simulink library "EngineSystemSubmodel"  (Simulink 8.1)
settings: Solver=ode45  StartTime=0.0  StopTime=10.0  FixedStep=1e-4  RelTol=1e-3
values from neighbouring files (symbols this model uses):
  B = [B1;B2]    [GensetRespOptimiztion.m]    (also in GensetRespOptimiztionTorstein.m; Init8RTFLEX68D.m = 0.68; init_MVM.m = 0.127)
  beta = 0.75    [Init8RTFLEX68D.m]
  cAStartRef = 104.8    [Init8RTFLEX68D.m]
  coeffMechEff = [0.135;0.155]    [Init8RTFLEX68D.m]
  comp_eff_map = [0 0 0 0 0 0 0 0 0 0 0 0 ... (250000 elements, 500x500)]    [comp_map.mat]    (also in comp_mapABB A175-35L.mat)
  comp_flow_map = [0 0 0 0 0 0 0 0 0 0 0 0 ... (250000 elements, 500x500)]    [comp_map.mat]    (also in comp_mapABB A175-35L.mat)
  D_turb_wheel = TC.TC_map.turb.D_wheel    [init_MVM.m]
  dCALiftDown = cAVVDownRef(end) - cAVVDownRef(1)    [Init8RTFLEX68D.m]
  dCALiftTopRef = 63.5    [Init8RTFLEX68D.m]
  dCALiftUp = cAVVUpRef(end) - cAVVUpRef(1)    [Init8RTFLEX68D.m]
  Dp = 0.383    [Init8RTFLEX68D.m]
  Ds = 0.079    [Init8RTFLEX68D.m]
  Dv = 0.425    [Init8RTFLEX68D.m]
  eff_coeff = [-1.0889528323728;0.91854258409396;-0.10659748546926;                     0.21229452390244;-0.053186221596493;-0.005451194709834]    [Init8RTFLEX68D.m]
  eta_turb_max = TC.TC_map.turb.eff_max    [init_MVM.m]
  flow_coeff_turb = [-1.585326540339;-4.823836967181;1.5853156139822]    [Init8RTFLEX68D.m]    (also in init_MVM.m = TC.TC_map.turb.flow_fit_coeff)
  fs = 0.0683    [Init8RTFLEX68D.m]    (also in NOxProcessGUI.m = varargin{2}; initHybrid.m; initMV.m; init_MVM.m = 0.0682925799315)
  genset = generators(1)    [runTempCyl4S.m]
  J_tc = TC.SAE_map_comp.inertia    [init_MVM.m]
  jShaft = 0    [EngineSystemParameters.m]    (also in Init8RTFLEX68D.m = 323000)
  jTC = 2    [Init8RTFLEX68D.m]
  Kb = 1*ones(engines,1)    [initHybrid.m]    (also in initMV.m; init_MVM.m = 1; init_ele.m = 1)
  Kd = 20*ones(engines,1)    [initHybrid.m]    (also in initMV.m; init_MVM.m = 10; init_ele.m = 20)
  Ki = 20*ones(engines,1)    [initHybrid.m]    (also in initMV.m; init_MVM.m = 10; init_ele.m = 20)
  Kp = 20*ones(engines,1)    [initHybrid.m]    (also in initMV.m; init_MVM.m = 10; init_ele.m = 20)
  lambdaCrank = 0.5056    [Init8RTFLEX68D.m]
  liftMax = 0.17    [Init8RTFLEX68D.m]
  Load_amp = x(4) + xRef(i)    [GetErrGensetResp.m]    (also in runsimulation.m = 0.55; runsimulationRecovery.m = InitialLoad(jj) + LoadStep(ii))
  Load_bias = x(4)    [GetErrGensetResp.m]    (also in runsimulation.m = 0.15; runsimulationRecovery.m = InitialLoad(jj))
  Load_index = 1    [GetErrGensetResp.m]    (also in runsimulation.m; runsimulationRecovery.m)
  mqfCycMax = 9.5547e-2    (= 0.095547)    [Init8RTFLEX68D.m]
  N = x*noMol    [NOxProcessGUI.m]    (also in initHybrid.m = .1*ones(engines,1); initMV.m = .1*ones(engines,1); init_ele.m = 0.1)
  n288_rep = [0 222.054 444.108 666.162 888.216 1110.27 1332.324 1554.378 1776.432 1998.486 2220.54 2442.594 ... (500 elements, 1x500)]    [comp_map.mat]
  nPort = 28    [Init8RTFLEX68D.m]
  npr = length(pr_rep)    [Init8RTFLEX68D.m]    (also in initHybrid.m; initMV.m; init_MVM.m)
  nsp = length(n288_rep)    [Init8RTFLEX68D.m]    (also in initHybrid.m; initMV.m; init_MVM.m)
  nStroke = 2    [Init8RTFLEX68D.m]
  omegat0 = RPM_TC_initial/30*pi    [init_MVM.m]
  pr_rep = [1.01 1.0150249672 1.0200499344 1.0250749016 1.0300998688 1.035124836 1.0401498032 1.0451747704 1.0501997376 1.0552247048 1.060249672 1.0652746392 ... (500 elements, 1x500)]    [comp_map.mat]
  r = 0.035    [Init8RTFLEX68D.m]
  Start_time = 50    [GetErrGensetResp.m]    (also in runsimulation.m; runsimulationRecovery.m)
  stroke = 2.72    [Init8RTFLEX68D.m]
  T_load = 1    [GetErrGensetResp.m]    (also in runsimulation.m; runsimulationRecovery.m)
  T_ref_turb = TC.TC_map.turb.T_ref    [init_MVM.m]
  u0 = 0.2    [init_MVM.m]
  Uc_opt = TC.TC_map.turb.Uc_opt    [init_MVM.m]
  w = 0.021    [Init8RTFLEX68D.m]
  wasteGateMax = 10    [Init8RTFLEX68D.m]
  wasteGateMin = 0    [Init8RTFLEX68D.m]
  wiebePara = [0.07;0.57;3.05;11;24;56.3;1.5;1;0.7]    [Init8RTFLEX68D.m]
  X = 0.07    [Init8RTFLEX68D.m]
  Y = 0.16    [Init8RTFLEX68D.m]
undefined symbols (not defined in the file or in its folder): aCrank, cAVVDownRef, cAVVUpRef, liftDownRef, liftUpRef, omega0, Td, Ti, u_max
undefined symbols (not defined in the file): BWdmExhBypass, cAlpha, cCylHT, E0A, ECyl0, hn, KbWG, KpWG, lowerCloseSPWG, m0A, mb0A, mbCyl0, mCp, mCyl0, nCyl, phi0, phi0A, phi0rad, RPM0, RPMMax, RPMT0, TiWG, upperOpenWG, V0A, vCyl0, wasteGateRatio
libraries: EngineSystemSubmodel x49, simulink x1
(part 3 of 3)

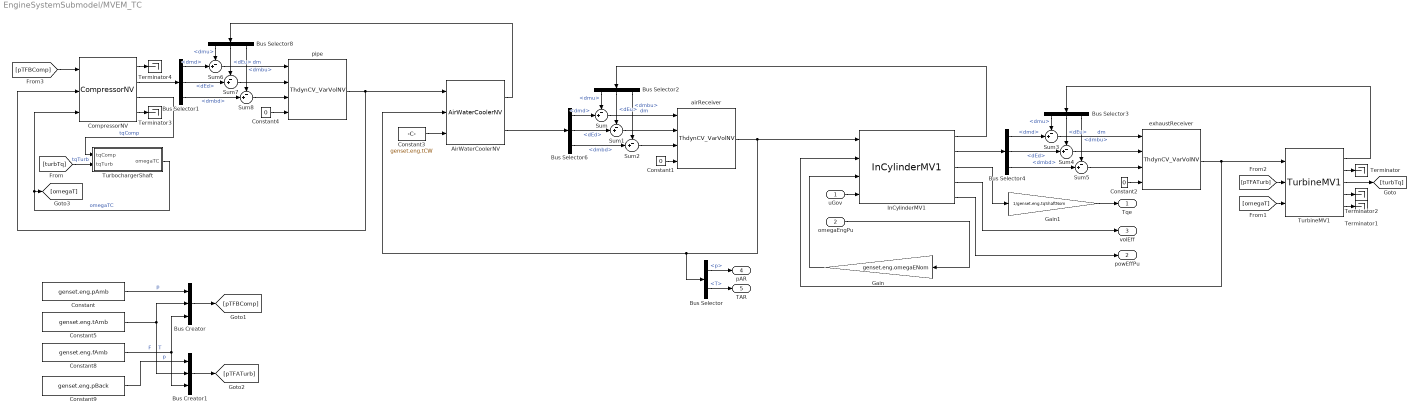
== system EngineSystemSubmodel/MVEM_TC ==
  uGov : Inport
  omegaEngPu : Inport  Port=2
  AirWaterCoolerNV : EngineSystemSubmodel/AirWaterCoolerNV  fs=genset.eng.fs  Cd=genset.eng.cdCool  A_air_path=genset.eng.aAirPath  dm_cw=genset.eng.dmCW  coeff_T_cw_K=genset.eng.coeffKTCW  Cp_cw=genset.eng.cpCW  D_cw_pipe=genset.eng.dPipeCW
  Bus Creator : BusCreator  Inputs=3
  Bus Creator1 : BusCreator  Inputs=3
  Bus Selector : BusSelector  OutputSignals=p,T
  Bus Selector1 : BusSelector  OutputSignals=dmd,dEd,dmbd
  Bus Selector2 : BusSelector  OutputSignals=dmu,dEu,dmbu
  Bus Selector3 : BusSelector  OutputSignals=dmu,dEu,dmbu
  Bus Selector4 : BusSelector  OutputSignals=dmd,dEd,dmbd
  Bus Selector6 : BusSelector  OutputSignals=dmd,dEd,dmbd
  Bus Selector8 : BusSelector  OutputSignals=dmu,dEu,dmbu
  CompressorNV : EngineSystemSubmodel/CompressorNV  fs=genset.eng.fs  comp_flow_map=genset.eng.compFlowMap  comp_eff_map=genset.eng.compEffMap  pr_rep=genset.eng.prRep  n288_rep=genset.eng.n288Rep  npr=genset.eng.npr  nsp=genset.eng.nsp
  Constant : Constant  Value=genset.eng.pAmb
  Constant1 : Constant  Value=0
  Constant2 : Constant  Value=0
  Constant3 : Constant  Value=genset.eng.tCW
  Constant4 : Constant  Value=0
  Constant5 : Constant  Value=genset.eng.tAmb
  Constant8 : Constant  Value=genset.eng.fAmb
  Constant9 : Constant  Value=genset.eng.pBack
  Gain : Gain  Gain=genset.eng.omegaENom
  Gain1 : Gain  Gain=1/genset.eng.tqShaftNom
  InCylinderMV1 : EngineSystemSubmodel/InCylinderMV1  fs=genset.eng.fs  Vd=genset.eng.vD  LHV=genset.eng.LHV  Pe_nom=genset.eng.powNom  SFC=genset.eng.SFC  vol_eff_coeff1=genset.eng.volEff1  vol_eff_coeff2=genset.eng.volEff2  T_pe=genset.eng.tPe  nstroke=genset.eng.nStroke  m_f_cyc_max=genset.eng.mFCycMax  C1=genset.eng.C1  p_a_inf=genset.eng.pAInf  Pe0=genset.eng.powL0*genset.eng.powNom
  Sum{,1..8} (9 alike) : Sum  Inputs=-+|
  Terminator{,1..4} (5 alike) : Terminator
  TurbineMV1 : EngineSystemSubmodel/TurbineMV1  fs=genset.eng.fs  flow_coeff_turb=genset.eng.flowCoeffTurb  D_turb_wheel=genset.eng.dTurbWheel  Uc_opt=genset.eng.ucOpt  eta_turb_max=genset.eng.effTurbMax  T_ref_turb=genset.eng.T_ref_turb
  TurbochargerShaft : Subsystem
  airReceiver : EngineSystemSubmodel/ThdynCV_VarVolNV  fs=genset.eng.fs  m0=genset.eng.m0AR  E0=genset.eng.E0AR  mb0=genset.eng.mb0AR  V0=genset.eng.vAR
  exhaustReceiver : EngineSystemSubmodel/ThdynCV_VarVolNV  fs=genset.eng.fs  m0=genset.eng.m0ER  E0=genset.eng.E0ER  mb0=genset.eng.mb0ER  V0=genset.eng.vER
  pipe : EngineSystemSubmodel/ThdynCV_VarVolNV  fs=genset.eng.fs  m0=genset.eng.m0PipeAComp  E0=genset.eng.e0PipeAComp  mb0=genset.eng.mb0PipeAComp  V0=genset.eng.vPipeAComp
  Tqe : Outport
  powEffPu : Outport  Port=2
  volEff : Outport  Port=3
  pAR : Outport  Port=4
  TAR : Outport  Port=5
  wires:
  TurbineMV1/2 -> Terminator/1
  TurbineMV1/4 -> Terminator2/1
  TurbineMV1/5 -> Terminator1/1
  Constant5/1 -> Bus Creator1/2, Bus Creator/2  "T"
  Constant8/1 -> Bus Creator1/3, Bus Creator/3  "F"
  Constant/1 -> Bus Creator/1  "p"
  Bus Creator1/1 -> [pTFATurb]
  Constant9/1 -> Bus Creator1/1  "p"
  Bus Selector3/2 -> Sum4/1  "<dEu>"
  [pTFBComp] -> CompressorNV/1
  [pTFATurb] -> TurbineMV1/2
  TurbineMV1/3 -> [turbTq]
  Bus Selector3/3 -> Sum5/1  "<dmbu>"
  InCylinderMV1/1 -> Bus Selector2/1
  Bus Selector2/1 -> Sum/1  "<dmu>"
  Sum/1 -> airReceiver/1  "dm"
  Bus Selector2/2 -> Sum1/1  "<dEu>"
  Bus Selector2/3 -> Sum2/1  "<dmbu>"
  exhaustReceiver/1 -> TurbineMV1/1, InCylinderMV1/2
  omegaEngPu/1 -> Gain/1
  airReceiver/1 -> InCylinderMV1/1, Bus Selector/1, AirWaterCoolerNV/2
  Constant4/1 -> pipe/4
  Bus Selector1/2 -> Sum7/2  "<dEd>"
  Bus Selector1/3 -> Sum8/2  "<dmbd>"
  Bus Selector1/1 -> Sum6/2  "<dmd>"
  Bus Creator/1 -> [pTFBComp]
  Bus Selector3/1 -> Sum3/1  "<dmu>"
  [omegaT] -> TurbineMV1/3
  TurbineMV1/1 -> Bus Selector3/1
  InCylinderMV1/5 -> powEffPu/1
  Sum6/1 -> pipe/1  "dm"
  AirWaterCoolerNV/2 -> Bus Selector6/1
  Bus Selector8/2 -> Sum7/1  "<dEu>"
  Sum7/1 -> pipe/2
  Bus Selector8/1 -> Sum6/1  "<dmu>"
  Gain/1 -> InCylinderMV1/3
  Sum8/1 -> pipe/3
  pipe/1 -> CompressorNV/2, AirWaterCoolerNV/1
  Bus Selector8/3 -> Sum8/1  "<dmbu>"
  AirWaterCoolerNV/1 -> Bus Selector8/1
  Bus Selector6/1 -> Sum/2  "<dmd>"
  Bus Selector6/2 -> Sum1/2  "<dEd>"
  Sum3/1 -> exhaustReceiver/1  "dm"
  Constant2/1 -> exhaustReceiver/4
  Sum5/1 -> exhaustReceiver/3
  Sum1/1 -> airReceiver/2
  Sum2/1 -> airReceiver/3
  Bus Selector4/2 -> Sum4/2  "<dEd>"
  Sum4/1 -> exhaustReceiver/2
  InCylinderMV1/2 -> Bus Selector4/1
  Bus Selector6/3 -> Sum2/2  "<dmbd>"
  Bus Selector4/3 -> Sum5/2  "<dmbd>"
  Constant1/1 -> airReceiver/4
  Bus Selector4/1 -> Sum3/2  "<dmd>"
  CompressorNV/2 -> Bus Selector1/1
  Constant3/1 -> AirWaterCoolerNV/3
  InCylinderMV1/4 -> volEff/1
  uGov/1 -> InCylinderMV1/4
  Gain1/1 -> Tqe/1
  Bus Selector/1 -> pAR/1  "<p>"
  Bus Selector/2 -> TAR/1  "<T>"
  CompressorNV/4 -> Terminator3/1
  CompressorNV/1 -> Terminator4/1
  InCylinderMV1/3 -> Gain1/1
  CompressorNV/3 -> TurbochargerShaft/1(tqComp)  "tqComp"
  [turbTq] -> TurbochargerShaft/2(tqTurb)  "tqTurb"
  TurbochargerShaft/1(omegaTC) -> CompressorNV/3, [omegaT]  "omegaTC"

== system EngineSystemSubmodel/ROHR ==
  pTF : Inport
  u_gov : Inport  Port=2
  phiInj : Inport  Port=3
  phi : Inport  Port=4
  omega : Inport  Port=5
  Demux : Demux  Outputs=3
  S-Function : S-Function  FunctionName=combState  Parameters=mqfCycMax,wiebePara  EnableBusSupport=off  mask{mqfCycMax=mqfCycMax, wiebePara=wiebePara}
      mask prompts: mqfCycMax "Maximum fuel mass injected per cycle [kg]"; wiebePara "3-Wiebe Parameters"
  S-Function1 : S-Function  FunctionName=CombWiebe  Parameters=hn, wiebePara  EnableBusSupport=off  mask{hn=hn, wiebePara=wiebePara}
      mask prompts: hn "Lower heating value of the fuel [J/kg]"; wiebePara "3-wiebe parameters"
  Terminator : Terminator
  dmEmb : Outport
  combState : Outport  Port=2
  phiIg : Outport  Port=3
  wires:
  S-Function/4 -> S-Function1/4  "mqf"
  S-Function/3 -> phiIg/1, S-Function1/3  "phiIg"
  S-Function/2 -> S-Function1/2  "phiComb"
  S-Function/1 -> S-Function1/1, combState/1  "combState"
  S-Function1/1 -> dmEmb/1
  Demux/3 -> Terminator/1
  Demux/2 -> S-Function/6  "T"
  Demux/1 -> S-Function/5  "p"
  pTF/1 -> Demux/1
  omega/1 -> S-Function/4, S-Function1/5
  u_gov/1 -> S-Function/3
  phiInj/1 -> S-Function/2
  phi/1 -> S-Function/1

== system EngineSystemSubmodel/Shaft ==
  tqEng : Inport
  tqLoad : Inport  Port=2
  Gain : Gain  Gain=HShaft  ParamDataTypeStr=double  OutDataTypeStr=double  mask{HShaft=HShaft}
      mask prompts: HShaft "Inverse of mass moment of inertia of the shaft (1/J) [kg-1m-2]"
  Integrator : Integrator  InitialCondition=jShaft*omegaE0  mask{jShaft=jShaft, omegaE0=omegaE0}
      mask prompts: jShaft "Mass moment of inertia of the shaft [kgm2]"; omegaE0 "Initial engine speed [rad/s]"
  MATLAB Function : MATLAB Function  TreatAsAtomicUnit=on  mask{omegaEMax=omegaEMax, coeffMechEff=coeffMechEff}
      mask prompts: omegaEMax "Maximum engine speed (rad/s)"; coeffMechEff "Coefficient for mechanical efficiency model (2x1)"
  Product : Product
  Sum : Sum  Inputs=|-+
  omegaE : Outport
  wires:
  tqLoad/1 -> Sum/1
  Integrator/1 -> Gain/1
  tqEng/1 -> Product/1
  MATLAB Function/1(effMech) -> Product/2  "effMech"
  Product/1 -> Sum/2  "TqShaft"
  Sum/1 -> Integrator/1
  Gain/1 -> MATLAB Function/1(omegaE), omegaE/1

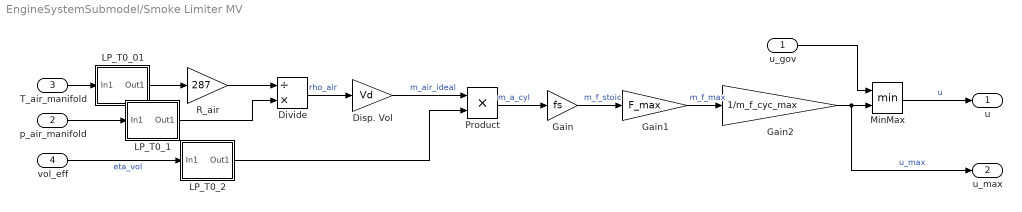
== system EngineSystemSubmodel/Smoke Limiter MV ==
  u_gov : Inport
  p_air_manifold : Inport  Port=2
  T_air_manifold : Inport  Port=3
  vol_eff : Inport  Port=4
  Disp. Vol : Gain  Gain=Vd
  Divide : Product  Inputs=/*
  Gain : Gain  Gain=fs
  Gain1 : Gain  Gain=F_max
  Gain2 : Gain  Gain=1/m_f_cyc_max
  LP_T0_01 : Subsystem
  LP_T0_1 : Subsystem
  LP_T0_2 : Subsystem
  MinMax : MinMax  Inputs=2
  Product : Product
  R_air : Gain  Gain=287
  u : Outport
  u_max : Outport  Port=2
  wires:
  LP_T0_2/1(Out1) -> Product/2
  LP_T0_1/1(Out1) -> Divide/2
  LP_T0_01/1(Out1) -> R_air/1
  Divide/1 -> Disp. Vol/1  "rho_air"
  p_air_manifold/1 -> LP_T0_1/1(In1)
  R_air/1 -> Divide/1
  T_air_manifold/1 -> LP_T0_01/1(In1)
  Disp. Vol/1 -> Product/1  "m_air_ideal"
  MinMax/1 -> u/1  "u"
  vol_eff/1 -> LP_T0_2/1(In1)  "eta_vol"
  Product/1 -> Gain/1  "m_a_cyl"
  u_gov/1 -> MinMax/1
  Gain/1 -> Gain1/1  "m_f_stoic"
  Gain1/1 -> Gain2/1  "m_f_max"
  Gain2/1 -> u_max/1, MinMax/2  "u_max"

== system EngineSystemSubmodel/SpeedController ==
  MV : Inport
  SP : Inport  Port=2
  Demux : Demux  Outputs=[1 ]
  Mux : Mux  Inputs=[1 1 ]
  S-Function : S-Function  FunctionName=SpeedController  Parameters=Kp,Td,N,Ti,max,min,u0  EnableBusSupport=off
  output : Outport
  wires:
  MV/1 -> Mux/1
  SP/1 -> Mux/2
  Demux/1 -> output/1
  Mux/1 -> S-Function/1
  S-Function/1 -> Demux/1

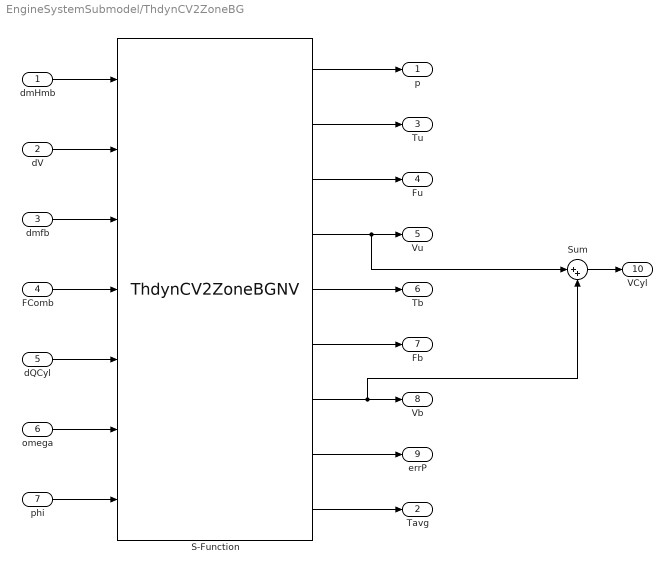
== system EngineSystemSubmodel/ThdynCV2ZoneBG ==
  dmHmb : Inport
  dV : Inport  Port=2
  dmfb : Inport  Port=3
  FComb : Inport  Port=4
  dQCyl : Inport  Port=5
  omega : Inport  Port=6
  phi : Inport  Port=7
  S-Function : S-Function  FunctionName=ThdynCV2ZoneBGNV  Parameters=fs, DPhiMix, phiMix0, alpha, hn, p0, T0, F0, V0  EnableBusSupport=off  mask{fs=fs, DPhiMix=DPhiMix, phiMix0=phiMix0, alpha=alpha, hn=hn, p0=p0, T0=T0, F0=F0, V0=V0}
      mask prompts: fs "Stoichiometric fuel-air ratio"; DPhiMix "Duration of mixing from burned zone to unburned zone [deg]"; phiMix0 "Start of mixing from burned zone to unburend [deg]"; alpha "Ratio of burned mass to unburned during gas exchange"; hn "Low heating value of the fuel [J/kg]"; p0 "Initial pressure [Pa]"; T0 "Initial temperature [K]"; F0 "Initial fuel-air equivalent ratio"; V0 "Initial volume [m3]"
  Sum : Sum  Inputs=|++
  p : Outport
  Tavg : Outport  Port=2
  Tu : Outport  Port=3
  Fu : Outport  Port=4
  Vu : Outport  Port=5
  Tb : Outport  Port=6
  Fb : Outport  Port=7
  Vb : Outport  Port=8
  errP : Outport  Port=9
  VCyl : Outport  Port=10
  wires:
  omega/1 -> S-Function/6
  S-Function/7 -> Sum/2, Vb/1
  dmHmb/1 -> S-Function/1
  dV/1 -> S-Function/2
  dQCyl/1 -> S-Function/5
  dmfb/1 -> S-Function/3
  S-Function/5 -> Tb/1
  S-Function/1 -> p/1
  FComb/1 -> S-Function/4
  phi/1 -> S-Function/7
  S-Function/2 -> Tu/1
  S-Function/4 -> Sum/1, Vu/1
  S-Function/3 -> Fu/1
  S-Function/8 -> errP/1
  S-Function/6 -> Fb/1
  S-Function/9 -> Tavg/1
  Sum/1 -> VCyl/1

== system EngineSystemSubmodel/ThdynCV_FixVol ==
  dmEmb : Inport
  Constant_V : Constant  Value=V
  Demux : Demux  Outputs=3
  Integrator_E : Integrator  InitialCondition=E0
  Integrator_m : Integrator  InitialCondition=m0
  Integrator_mb : Integrator  InitialCondition=mb0
  Mux : Mux  Inputs=3
  S-Function : S-Function  FunctionName=ThdynCV  Parameters=fs  SFunctionModules=GetThdynCombGasZach.c GetPTF.c  EnableBusSupport=off
  pTF : Outport
  wires:
  Demux/1 -> Integrator_m/1
  dmEmb/1 -> Demux/1
  Demux/2 -> Integrator_E/1
  Demux/3 -> Integrator_mb/1
  Integrator_m/1 -> S-Function/1
  Integrator_E/1 -> S-Function/2
  Integrator_mb/1 -> S-Function/3
  Constant_V/1 -> S-Function/4
  S-Function/3 -> Mux/3
  S-Function/1 -> Mux/1
  Mux/1 -> pTF/1
  S-Function/2 -> Mux/2

== system EngineSystemSubmodel/ThdynCV_VarVol ==
  dmEmb : Inport
  dV : Inport  Port=2
  Demux : Demux  Outputs=3
  Integrator_E : Integrator  InitialCondition=E0
  Integrator_V : Integrator  InitialCondition=V0
  Integrator_m : Integrator  InitialCondition=m0
  Integrator_mb : Integrator  InitialCondition=mb0
  Mux : Mux  Inputs=3
  S-Function : S-Function  FunctionName=ThdynCV  Parameters=fs  SFunctionModules=GetThdynCombGasZach.c GetPTF.c  EnableBusSupport=off
  pTF : Outport
  p : Outport  Port=2
  v : Outport  Port=3
  wires:
  Demux/1 -> Integrator_m/1
  dmEmb/1 -> Demux/1
  Demux/2 -> Integrator_E/1
  Demux/3 -> Integrator_mb/1
  Integrator_m/1 -> S-Function/1
  Integrator_E/1 -> S-Function/2
  Integrator_mb/1 -> S-Function/3
  dV/1 -> Integrator_V/1
  S-Function/1 -> p/1, Mux/1
  Mux/1 -> pTF/1
  S-Function/2 -> Mux/2
  Integrator_V/1 -> S-Function/4, v/1
  S-Function/3 -> Mux/3

== system EngineSystemSubmodel/ThdynCV_VarVolConv ==
  dmEmb : Inport
  dV : Inport  Port=2
  Demux : Demux  Outputs=3
  Mux : Mux  Inputs=3
  S-Function : S-Function  FunctionName=ThdynCVConv  Parameters=fs,p0,T0,F0,V0  EnableBusSupport=off  mask{fs=fs, p0=p0, T0=T0, F0=F0, V0=V0}
      mask prompts: fs "Stoichiometric fuel-air ratio"; p0 "Initial pressure"; T0 "Initial temperature"; F0 "Initial fuel-air equivalent ratio"; V0 "Initial volume"
  pTF : Outport
  p : Outport  Port=2
  V : Outport  Port=3
  wires:
  Demux/1 -> S-Function/1
  Demux/2 -> S-Function/2
  Demux/3 -> S-Function/3
  dmEmb/1 -> Demux/1
  dV/1 -> S-Function/4
  S-Function/2 -> Mux/2
  S-Function/3 -> Mux/3
  S-Function/4 -> V/1
  Mux/1 -> pTF/1
  S-Function/1 -> p/1, Mux/1

== system EngineSystemSubmodel/ThdynCV_VarVolNV ==
  dm : Inport
  dE : Inport  Port=2
  dmb : Inport  Port=3
  dV : Inport  Port=4
  Bus Creator : BusCreator
  S-Function : S-Function  FunctionName=ThdynCVNV  Parameters=fs,m0,E0,mb0,V0  SFunctionModules=GetThdynCombGasZach.c GetPTF.c  EnableBusSupport=off
  pTFV : Outport
  wires:
  dE/1 -> S-Function/2
  dm/1 -> S-Function/1
  dmb/1 -> S-Function/3
  dV/1 -> S-Function/4
  S-Function/2 -> Bus Creator/2  "T"
  S-Function/1 -> Bus Creator/1  "p"
  S-Function/3 -> Bus Creator/3  "F"
  S-Function/4 -> Bus Creator/4  "V"
  Bus Creator/1 -> pTFV/1

== system EngineSystemSubmodel/Turbine ==
  pTF_u : Inport
  pTF_d : Inport  Port=2
  omegat : Inport  Port=3
  Demux : Demux  Outputs=3
  Demux1 : Demux  Outputs=3
  Mux : Mux  Inputs=3
  Mux1 : Mux  Inputs=3
  S-Function : S-Function  FunctionName=turbine_calc_PTF  Parameters=fs,flow_coeff_turb,eff_coeff  SFunctionModules=GetThdynCombGasZach.c  EnableBusSupport=off  mask{fs=fs, flow_coeff_turb=flow_coeff_turb, eff_coeff=eff_coeff}
      mask prompts: fs "Stoichiometric fuel air ratio"; flow_coeff_turb "Coefficient for flow model of turbine"; eff_coeff "Coefficient for efficiency model of turbine"
  dmEmb_u : Outport
  dmEmb_d : Outport  Port=2
  Tqt : Outport  Port=3
  Td_calc : Outport  Port=4
  effTurb : Outport  Port=5
  wires:
  Demux/1 -> S-Function/1
  Demux/3 -> S-Function/3
  Demux/2 -> S-Function/2
  Demux1/2 -> S-Function/5
  Demux1/3 -> S-Function/6
  Demux1/1 -> S-Function/4
  pTF_d/1 -> Demux1/1
  omegat/1 -> S-Function/7
  pTF_u/1 -> Demux/1
  S-Function/8 -> Td_calc/1
  S-Function/5 -> Mux1/2
  S-Function/4 -> Mux1/1
  S-Function/6 -> Mux1/3
  S-Function/1 -> Mux/1
  S-Function/2 -> Mux/2
  S-Function/3 -> Mux/3
  Mux/1 -> dmEmb_u/1
  Mux1/1 -> dmEmb_d/1
  S-Function/7 -> Tqt/1
  S-Function/9 -> effTurb/1

== system EngineSystemSubmodel/TurbineMV ==
  pTF_u : Inport
  pTF_d : Inport  Port=2
  omegat : Inport  Port=3
  Demux : Demux  Outputs=3
  Demux1 : Demux  Outputs=3
  Mux : Mux  Inputs=3
  Mux1 : Mux  Inputs=3
  S-Function : S-Function  FunctionName=turbine_calc_MV_PTF  Parameters=fs,flow_coeff_turb,D_turb_wheel,Uc_opt,eta_turb_max,T_ref_turb  SFunctionModules=GetThdynCombGasZach.c  EnableBusSupport=off
  dmEmb_u : Outport
  dmEmb_d : Outport  Port=2
  Tqt : Outport  Port=3
  Td_calc : Outport  Port=4
  eta_t : Outport  Port=5
  wires:
  Demux/1 -> S-Function/1
  Demux/3 -> S-Function/3
  Demux/2 -> S-Function/2
  Demux1/2 -> S-Function/5
  Demux1/3 -> S-Function/6
  Demux1/1 -> S-Function/4
  pTF_d/1 -> Demux1/1
  omegat/1 -> S-Function/7
  pTF_u/1 -> Demux/1
  S-Function/8 -> Td_calc/1
  S-Function/5 -> Mux1/2
  S-Function/4 -> Mux1/1
  S-Function/6 -> Mux1/3
  S-Function/1 -> Mux/1
  S-Function/2 -> Mux/2
  S-Function/3 -> Mux/3
  Mux/1 -> dmEmb_u/1
  Mux1/1 -> dmEmb_d/1
  S-Function/7 -> Tqt/1
  S-Function/9 -> eta_t/1

== system EngineSystemSubmodel/TurbineMV1 ==
  pTF_u : Inport
  pTF_d : Inport  Port=2
  omegat : Inport  Port=3
  Bus Creator : BusCreator  Inputs=3
  Bus Creator1 : BusCreator  Inputs=3
  Bus Selector : BusSelector  OutputSignals=p,T,F
  Bus Selector1 : BusSelector  OutputSignals=p,T,F
  S-Function : S-Function  FunctionName=turbine_calc_MV_PTF  Parameters=fs,flow_coeff_turb,D_turb_wheel,Uc_opt,eta_turb_max,T_ref_turb  SFunctionModules=GetThdynCombGasZach.c  EnableBusSupport=off
  dmEmb_u : Outport
  dmEmb_d : Outport  Port=2
  Tqt : Outport  Port=3
  Td_calc : Outport  Port=4
  eta_t : Outport  Port=5
  wires:
  pTF_u/1 -> Bus Selector/1
  Bus Selector/2 -> S-Function/2  "<T>"
  Bus Selector/3 -> S-Function/3  "<F>"
  Bus Selector/1 -> S-Function/1  "<p>"
  pTF_d/1 -> Bus Selector1/1
  Bus Selector1/2 -> S-Function/5  "<T>"
  Bus Selector1/3 -> S-Function/6  "<F>"
  Bus Selector1/1 -> S-Function/4  "<p>"
  omegat/1 -> S-Function/7
  S-Function/1 -> Bus Creator/1  "dmu"
  S-Function/2 -> Bus Creator/2  "dEu"
  S-Function/3 -> Bus Creator/3  "dmbu"
  Bus Creator/1 -> dmEmb_u/1
  S-Function/4 -> Bus Creator1/1  "dmd"
  S-Function/5 -> Bus Creator1/2  "dEd"
  S-Function/6 -> Bus Creator1/3  "dmbd"
  Bus Creator1/1 -> dmEmb_d/1
  S-Function/7 -> Tqt/1
  S-Function/8 -> Td_calc/1
  S-Function/9 -> eta_t/1

== system EngineSystemSubmodel/Turbocharger ==
  pTF_c_u : Inport
  pTF_c_d : Inport  Port=2
  pTF_t_u : Inport  Port=3
  pTF_t_d : Inport  Port=4
  Compressor1 : EngineSystemSubmodel/Compressor  fs=fs  comp_flow_map=comp_flow_map  comp_eff_map=comp_eff_map  pr_rep=pr_rep  n288_rep=n288_rep  npr=npr  nsp=nsp
  Constant : Constant  Value=jTC
  Integrator : Integrator  InitialCondition=omegat0*jTC
  Product : Product  Inputs=*/
  Sum : Sum  Inputs=-|+
  Terminator : Terminator
  Terminator1 : Terminator
  Turbine1 : EngineSystemSubmodel/Turbine  fs=fs  flow_coeff_turb=flow_coeff_turb  eff_coeff=eff_coeff
  dmEmb_c_u : Outport
  dmEmb_c_d : Outport  Port=2
  dmEmb_t_u : Outport  Port=3
  dmEmb_t_d : Outport  Port=4
  T_t_d_calc : Outport  Port=5
  wires:
  pTF_c_d/1 -> Compressor1/2
  Turbine1/3 -> Sum/2  "tqTurb"
  Turbine1/1 -> dmEmb_t_u/1
  Compressor1/1 -> dmEmb_c_u/1
  Product/1 -> Turbine1/3, Compressor1/3  "omegat"
  Compressor1/2 -> dmEmb_c_d/1
  Integrator/1 -> Product/1
  Sum/1 -> Integrator/1
  Compressor1/3 -> Sum/1  "tqComp"
  Turbine1/2 -> dmEmb_t_d/1
  Turbine1/4 -> T_t_d_calc/1  "tempATurb"
  pTF_c_u/1 -> Compressor1/1
  pTF_t_u/1 -> Turbine1/1
  pTF_t_d/1 -> Turbine1/2
  Constant/1 -> Product/2
  Compressor1/4 -> Terminator/1  "effComp"
  Turbine1/5 -> Terminator1/1  "effTurb"

== system EngineSystemSubmodel/TurbochargerMV ==
  pTF_c_u : Inport
  pTF_c_d : Inport  Port=2
  pTF_t_u : Inport  Port=3
  pTF_t_d : Inport  Port=4
  Compressor : EngineSystemSubmodel/Compressor  fs=fs  comp_flow_map=comp_flow_map  comp_eff_map=comp_eff_map  pr_rep=pr_rep  n288_rep=n288_rep  npr=npr  nsp=nsp
  Gain : Gain  Gain=1/J_tc
  Integrator : Integrator  InitialCondition=omegat0*J_tc
  Sum : Sum  Inputs=-|+
  TurbineMV : EngineSystemSubmodel/TurbineMV  fs=fs  flow_coeff_turb=flow_coeff_turb  D_turb_wheel=D_turb_wheel  Uc_opt=Uc_opt  eta_turb_max=eta_turb_max
  dmEmb_c_u : Outport
  dmEmb_c_d : Outport  Port=2
  dmEmb_t_u : Outport  Port=3
  dmEmb_t_d : Outport  Port=4
  T_t_d_calc : Outport  Port=5
  eta_c : Outport  Port=6
  eta_t : Outport  Port=7
  wires:
  TurbineMV/5 -> eta_t/1
  TurbineMV/3 -> Sum/2  "Tqt"
  TurbineMV/1 -> dmEmb_t_u/1
  Compressor/1 -> dmEmb_c_u/1
  Gain/1 -> Compressor/3, TurbineMV/3  "omegat"
  Compressor/2 -> dmEmb_c_d/1
  Integrator/1 -> Gain/1
  Sum/1 -> Integrator/1
  Compressor/3 -> Sum/1  "Tqc"
  TurbineMV/2 -> dmEmb_t_d/1
  TurbineMV/4 -> T_t_d_calc/1
  pTF_c_d/1 -> Compressor/2
  pTF_c_u/1 -> Compressor/1
  pTF_t_u/1 -> TurbineMV/1
  pTF_t_d/1 -> TurbineMV/2
  Compressor/4 -> eta_c/1

== system EngineSystemSubmodel/TurbochargerMV1 ==
  pTF_c_u : Inport
  pTF_c_d : Inport  Port=2
  pTF_t_u : Inport  Port=3
  pTF_t_d : Inport  Port=4
  Compressor : EngineSystemSubmodel/Compressor  fs=fs  comp_flow_map=comp_flow_map  comp_eff_map=comp_eff_map  pr_rep=pr_rep  n288_rep=n288_rep  npr=npr  nsp=nsp
  Gain : Gain  Gain=1/J_tc
  Integrator : Integrator  InitialCondition=omegat0*J_tc
  Sum : Sum  Inputs=-|+
  TurbineMV : EngineSystemSubmodel/TurbineMV  fs=fs  flow_coeff_turb=flow_coeff_turb  D_turb_wheel=D_turb_wheel  Uc_opt=Uc_opt  eta_turb_max=eta_turb_max
  dmEmb_c_u : Outport
  dmEmb_c_d : Outport  Port=2
  dmEmb_t_u : Outport  Port=3
  dmEmb_t_d : Outport  Port=4
  T_t_d_calc : Outport  Port=5
  eta_c : Outport  Port=6
  eta_t : Outport  Port=7
  wires:
  TurbineMV/5 -> eta_t/1
  TurbineMV/3 -> Sum/2  "Tqt"
  TurbineMV/1 -> dmEmb_t_u/1
  Compressor/1 -> dmEmb_c_u/1
  Gain/1 -> Compressor/3, TurbineMV/3  "omegat"
  Compressor/2 -> dmEmb_c_d/1
  Integrator/1 -> Gain/1
  Sum/1 -> Integrator/1
  Compressor/3 -> Sum/1  "Tqc"
  TurbineMV/2 -> dmEmb_t_d/1
  TurbineMV/4 -> T_t_d_calc/1
  pTF_c_d/1 -> Compressor/2
  pTF_c_u/1 -> Compressor/1
  pTF_t_u/1 -> TurbineMV/1
  pTF_t_d/1 -> TurbineMV/2
  Compressor/4 -> eta_c/1

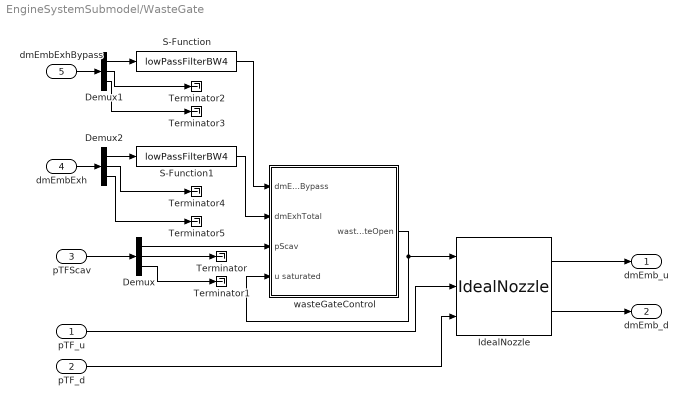
== system EngineSystemSubmodel/WasteGate ==
  pTF_u : Inport
  pTF_d : Inport  Port=2
  pTFScav : Inport  Port=3
  dmEmbExh : Inport  Port=4
  dmEmbExhBypass : Inport  Port=5
  Demux : Demux  Outputs=3
  Demux1 : Demux  Outputs=3
  Demux2 : Demux  Outputs=3
  IdealNozzle : EngineSystemSubmodel/IdealNozzle  fs=fs
  S-Function : S-Function  FunctionName=lowPassFilterBW4  Parameters=BW,y0  EnableBusSupport=off  mask{BW=BWdmExhBypass, y0=0}
      mask prompts: BW "Bandwidth [Hz]"; y0 "Initial output"
  S-Function1 : S-Function  FunctionName=lowPassFilterBW4  Parameters=BW,y0  EnableBusSupport=off  mask{BW=BWdmExh, y0=0}
      mask prompts: BW "Bandwidth [Hz]"; y0 "Initial output"
  Terminator{,1..5} (6 alike) : Terminator
  wasteGateControl : Subsystem  mask{Kp=Kp, Ti=Ti, K_b=K_b, max=max, min=min, bypassRatio=bypassRatio, upper=upper, lower=lower}
      mask prompts: Kp "Proportional gain"; Ti "Integral time constant"; K_b "Back calculation gain for anti-windup"; max "Maximum allowable valve opening"; min "Maximum allowable valve opening"; bypassRatio "Bypass ratio"; upper "Upper bound for opening waste gate"; lower "Lower bound for closing waste gate"
      mask TypeOptions Kp: Gain/Kp | Gain2/Kp
      mask TypeOptions Ti: Gain1/Ti
      mask TypeOptions K_b: Gain3/K_b
      mask TypeOptions max: Saturation/max
      mask TypeOptions min: Saturation/min
      mask TypeOptions bypassRatio: Constant1/bypassRatio
      mask TypeOptions upper: S-Function/upper
      mask TypeOptions lower: S-Function/lower
  dmEmb_u : Outport
  dmEmb_d : Outport  Port=2
  wires:
  Demux2/3 -> Terminator5/1
  Demux2/2 -> Terminator4/1
  Demux2/1 -> S-Function1/1
  dmEmbExh/1 -> Demux2/1
  Demux1/3 -> Terminator3/1
  Demux1/2 -> Terminator2/1
  Demux1/1 -> S-Function/1
  dmEmbExhBypass/1 -> Demux1/1
  Demux/3 -> Terminator1/1
  Demux/2 -> Terminator/1
  Demux/1 -> wasteGateControl/3(pScav)
  S-Function/1 -> wasteGateControl/1(dmExhBypass)
  pTFScav/1 -> Demux/1
  S-Function1/1 -> wasteGateControl/2(dmExhTotal)
  pTF_d/1 -> IdealNozzle/3
  pTF_u/1 -> IdealNozzle/2
  wasteGateControl/1(wasteGateOpen) -> IdealNozzle/1, wasteGateControl/4(u saturated)
  IdealNozzle/1 -> dmEmb_u/1
  IdealNozzle/2 -> dmEmb_d/1

== system EngineSystemSubmodel/pMaxFinder ==
  phi : Inport
  pCyl : Inport  Port=2
  Clock : Clock
      settings: Decimation=6
  S-Function : S-Function  FunctionName=pMaxFinder  EnableBusSupport=off
  pMax : Outport
  phiAtPMax : Outport  Port=2
  wires:
  S-Function/2 -> phiAtPMax/1
  S-Function/1 -> pMax/1
  pCyl/1 -> S-Function/3
  phi/1 -> S-Function/2
  Clock/1 -> S-Function/1

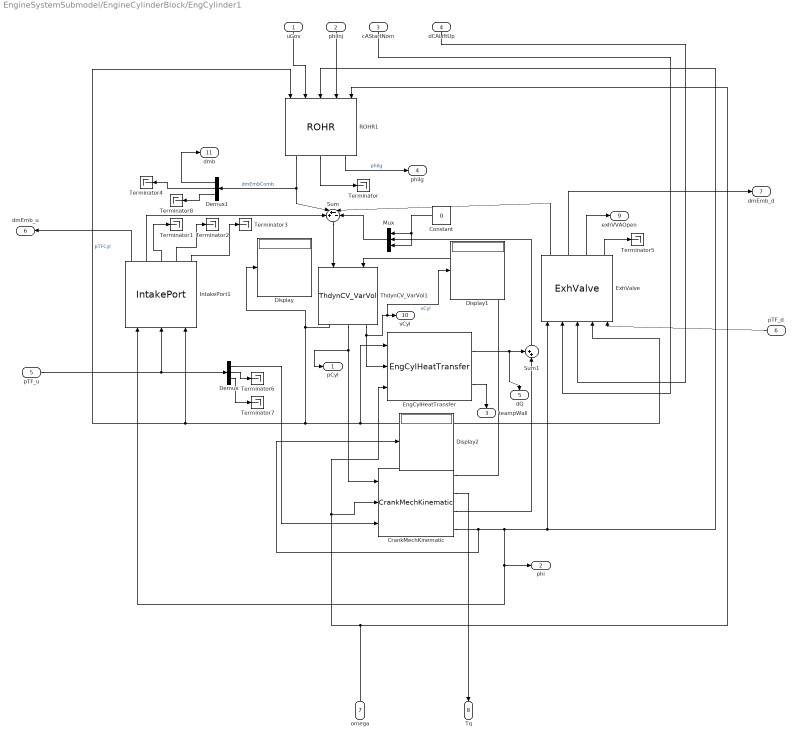
== system EngineSystemSubmodel/EngineCylinderBlock/EngCylinder1 ==
  uGov : Inport
  phiInj : Inport  Port=2
  cAStartNom : Inport  Port=3
  dCALiftUp : Inport  Port=4
  pTF_u : Inport  Port=5
  pTF_d : Inport  Port=6
  omega : Inport  Port=7
  Constant : Constant  Value=0
  CrankMechKinematic : EngineSystemSubmodel/CrankMechKinematic  phi0=phi0  B=B  stroke=stroke  lambdaCrank=lambdaCrank
  Demux : Demux  Outputs=3
  Demux1 : Demux  Outputs=3
  Display : Display
  Display1 : Display
  Display2 : Display
  EngCylHeatTransfer : EngineSystemSubmodel/EngCylHeatTransfer  stroke=stroke  B=B  cAlpha=cAlpha  mCp=mCp  cCylHT=cCylHT  nCyl=nCyl  tempWall0=600
  ExhValve : EngineSystemSubmodel/ExhValve  fs=fs  cAVVUpRef=cAVVUpRef  cAVVDownRef=cAVVDownRef  liftUpRef=liftUpRef  liftDownRef=liftDownRef  cAStartRef=cAStartRef  dCALiftUp=dCALiftUp  dCALiftDown=dCALiftDown  dCALiftTopRef=dCALiftTopRef  liftMax=liftMax  Dv=Dv  beta=beta  w=w  Dp=Dp  Ds=Ds
  IntakePort1 : EngineSystemSubmodel/IntakePort  fs=fs  nStroke=nStroke  aCrank=aCrank  lambdaCrank=lambdaCrank  X=X  Y=Y  r=r  nPort=nPort  stroke=stroke
  Mux : Mux  Inputs=3
  ROHR1 : EngineSystemSubmodel/ROHR  mqfCycMax=mqfCycMax  wiebePara=wiebePara  hn=hn
  Sum : Sum  Inputs=++--
  Sum1 : Sum  Inputs=++|
  Terminator{,1..8} (9 alike) : Terminator
  ThdynCV_VarVol1 : EngineSystemSubmodel/ThdynCV_VarVol  fs=fs  m0=m0  E0=E0  mb0=mb0  V0=V0
  pCyl : Outport
  phi : Outport  Port=2
  teampWall : Outport  Port=3
  phiIg : Outport  Port=4
  dQ : Outport  Port=5
  dmEmb_u : Outport  Port=6
  dmEmb_d : Outport  Port=7
  Tq : Outport  Port=8
  exhVVAOpen : Outport  Port=9
  vCyl : Outport  Port=10
  dmb : Outport  Port=11
  wires:
  Demux1/3 -> Terminator8/1
  Demux1/2 -> Terminator4/1
  Demux1/1 -> dmb/1
  ROHR1/3 -> phiIg/1  "phiIg"
  EngCylHeatTransfer/2 -> teampWall/1
  Demux/3 -> Terminator7/1
  Demux/2 -> Terminator6/1
  Constant/1 -> Mux/1, Mux/3
  Mux/1 -> Sum/4
  Sum1/1 -> Mux/2
  EngCylHeatTransfer/1 -> dQ/1, Sum1/1
  ThdynCV_VarVol1/3 -> EngCylHeatTransfer/2, Display1/1, vCyl/1  "vCyl"
  ExhValve/2 -> dmEmb_d/1
  IntakePort1/4 -> Terminator2/1
  pTF_u/1 -> Demux/1, IntakePort1/2
  ExhValve/3 -> exhVVAOpen/1
  IntakePort1/5 -> Terminator3/1
  dCALiftUp/1 -> ExhValve/3
  IntakePort1/3 -> Terminator1/1
  IntakePort1/1 -> dmEmb_u/1
  ROHR1/2 -> Terminator/1
  omega/1 -> CrankMechKinematic/2, EngCylHeatTransfer/3, ROHR1/5
  pTF_d/1 -> ExhValve/5
  phiInj/1 -> ROHR1/4
  CrankMechKinematic/2 -> Tq/1
  Demux/1 -> CrankMechKinematic/3
  ExhValve/4 -> Terminator5/1
  CrankMechKinematic/3 -> Sum1/2
  uGov/1 -> ROHR1/2
  cAStartNom/1 -> ExhValve/2
  CrankMechKinematic/1 -> ThdynCV_VarVol1/2
  ThdynCV_VarVol1/2 -> pCyl/1, CrankMechKinematic/1
  ThdynCV_VarVol1/1 -> IntakePort1/3, ROHR1/1, ExhValve/4, EngCylHeatTransfer/1, Display/1  "pTFCyl"
  Sum/1 -> ThdynCV_VarVol1/1
  ROHR1/1 -> Sum/2, Demux1/1  "dmEmbComb"
  ExhValve/1 -> Sum/3
  IntakePort1/2 -> Sum/1
  CrankMechKinematic/4 -> Display2/1, IntakePort1/1, phi/1, ExhValve/1, ROHR1/3

== system EngineSystemSubmodel/Governor/PID controller ==
  e : Inport  PortDimensions=1
  omega_pu : Inport  Port=2  PortDimensions=1
  u saturated : Inport  Port=3  PortDimensions=1
  D : Gain  DisableCoverage=on  Gain=genset.governor.N
  Filter : Integrator  DisableCoverage=on  InitialCondition=-genset.omega0*genset.governor.Kd
  Gain2 : Gain  Gain=-genset.governor.Kd
  I : Gain  Gain=genset.governor.Ki
  Integrator : Integrator  DisableCoverage=on  InitialCondition=genset.u0
  Kb : Gain  DisableCoverage=on  Gain=genset.governor.Kb  ParamDataTypeStr=Inherit: Inherit from 'Gain'
  P : Gain  Gain=genset.governor.Kp
  Saturation : Saturate  UpperLimit=genset.u_max  LowerLimit=genset.u_min  LinearizeAsGain=off  OutMin=genset.u_min  OutMax=genset.u_max  OutDataTypeStr=Inherit: Inherit via back propagation
  Sum1 : Sum  Inputs=+++
  SumD : Sum  DisableCoverage=on  Inputs=|+-
  SumI1 : Sum  DisableCoverage=on  Inputs=|++
  SumI2 : Sum  DisableCoverage=on  Inputs=-+|
  u : Outport  PortDimensions=1  InitialOutput=0
  wires:
  I/1 -> Integrator/1
  SumI1/1 -> I/1
  u saturated/1 -> SumI2/2
  Kb/1 -> SumI1/2
  SumI2/1 -> Kb/1  "u_sat_error"
  Sum1/1 -> SumI2/1, Saturation/1
  Gain2/1 -> SumD/1
  SumD/1 -> D/1
  Filter/1 -> SumD/2  "xid"
  Saturation/1 -> u/1
  P/1 -> Sum1/1  "governor_P"
  e/1 -> SumI1/1, P/1  "err_governor"
  omega_pu/1 -> Gain2/1
  D/1 -> Filter/1, Sum1/2  "governor_D"
  Integrator/1 -> Sum1/3  "governor_I"

== system EngineSystemSubmodel/Governor_SpeedControl/PID controller ==
  e : Inport  PortDimensions=1
  omega_pu : Inport  Port=2  PortDimensions=1
  u saturated : Inport  Port=3  PortDimensions=1
  D : Gain  DisableCoverage=on  Gain=N
  Filter : Integrator  DisableCoverage=on  InitialCondition=-omega0*Kd
  Gain2 : Gain  Gain=Kd
  I : Gain  Gain=Ki
  Integrator : Integrator  DisableCoverage=on  InitialCondition=u0
  Kb : Gain  DisableCoverage=on  Gain=Kb  ParamDataTypeStr=Inherit: Inherit from 'Gain'
  P : Gain  Gain=Kp
  Saturation : Saturate  UpperLimit=u_max  LowerLimit=u_min  LinearizeAsGain=off  OutMin=u_min  OutMax=u_max  OutDataTypeStr=Inherit: Inherit via back propagation
  Sum1 : Sum  Inputs=+++
  SumD : Sum  DisableCoverage=on  Inputs=|+-
  SumI1 : Sum  DisableCoverage=on  Inputs=|++
  SumI2 : Sum  DisableCoverage=on  Inputs=-+|
  u : Outport  PortDimensions=1  InitialOutput=0
  wires:
  I/1 -> Integrator/1
  SumI1/1 -> I/1
  u saturated/1 -> SumI2/2
  Kb/1 -> SumI1/2
  SumI2/1 -> Kb/1  "u_sat_error"
  Sum1/1 -> SumI2/1, Saturation/1
  Gain2/1 -> SumD/1
  SumD/1 -> D/1
  Filter/1 -> SumD/2  "xid"
  Saturation/1 -> u/1
  P/1 -> Sum1/1  "governor_P"
  e/1 -> SumI1/1, P/1
  omega_pu/1 -> Gain2/1
  D/1 -> Filter/1, Sum1/2  "governor_D"
  Integrator/1 -> Sum1/3  "governor_I"

== system EngineSystemSubmodel/MVEM_TC/TurbochargerShaft ==
  tqComp : Inport
  tqTurb : Inport  Port=2
  Gain1 : Gain
  Gain3 : Gain  Gain=1/genset.eng.jTC
  Integrator : Integrator  InitialCondition=genset.eng.omegaT0*genset.eng.jTC
  Saturation : Saturate  UpperLimit=genset.eng.RPMtMax*pi/30*1.1;  LowerLimit=genset.eng.RPMtMax*pi/30*0.24;
  Sum10 : Sum  Inputs=-+|
  Sum9 : Sum  Inputs=-++
  omegaTC : Outport
  wires:
  tqComp/1 -> Sum9/1
  tqTurb/1 -> Sum9/2
  Sum9/1 -> Integrator/1
  Integrator/1 -> Gain3/1
  Gain3/1 -> Saturation/1, Sum10/1  "omegat"
  Sum10/1 -> Gain1/1
  Saturation/1 -> Sum10/2, omegaTC/1
  Gain1/1 -> Sum9/3

== system EngineSystemSubmodel/Smoke Limiter MV/LP_T0_01 ==
  In1 : Inport
  Gain3 : Gain  Gain=100
  Integrator : Integrator  InitialCondition=1
  Sum : Sum  Inputs=|+-
  Out1 : Outport
  wires:
  Integrator/1 -> Sum/2, Out1/1
  In1/1 -> Sum/1
  Sum/1 -> Gain3/1
  Gain3/1 -> Integrator/1

== system EngineSystemSubmodel/Smoke Limiter MV/LP_T0_1 ==
  In1 : Inport
  Gain3 : Gain  Gain=100
  Integrator : Integrator  InitialCondition=1
  Sum : Sum  Inputs=|+-
  Out1 : Outport
  wires:
  Integrator/1 -> Sum/2, Out1/1
  In1/1 -> Sum/1
  Sum/1 -> Gain3/1
  Gain3/1 -> Integrator/1

== system EngineSystemSubmodel/Smoke Limiter MV/LP_T0_2 ==
  In1 : Inport
  Gain3 : Gain  Gain=100
  Integrator : Integrator  InitialCondition=1
  Sum : Sum  Inputs=|+-
  Out1 : Outport
  wires:
  Integrator/1 -> Sum/2, Out1/1
  In1/1 -> Sum/1
  Sum/1 -> Gain3/1
  Gain3/1 -> Integrator/1

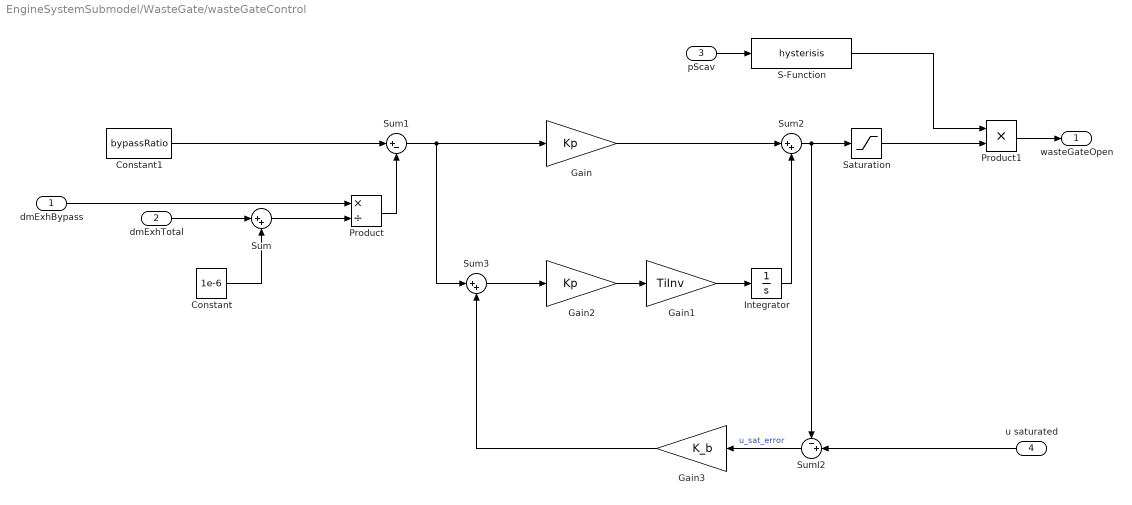
== system EngineSystemSubmodel/WasteGate/wasteGateControl ==
  dmExhBypass : Inport
  dmExhTotal : Inport  Port=2
  pScav : Inport  Port=3
  u saturated : Inport  Port=4  PortDimensions=1
  Constant : Constant  Value=1e-6
  Constant1 : Constant  Value=bypassRatio  mask{bypassRatio=bypassRatio}
      mask prompts: bypassRatio "Bypass ratio"
  Gain : Gain  Gain=Kp  mask{Kp=Kp}
      mask prompts: Kp "Proportional gain"
  Gain1 : Gain  Gain=TiInv  mask{Ti=Ti, TiInv=0}
      mask prompts: Ti "Integral time constant"; TiInv "Inverse of time constant"
      mask init:
      | TiInv = 1./Ti;
  Gain2 : Gain  Gain=Kp  mask{Kp=Kp}
      mask prompts: Kp "Proportional gain"
  Gain3 : Gain  Gain=K_b  mask{K_b=K_b}
      mask prompts: K_b "Back calculation gain for anti-windup"
  Integrator : Integrator  InitialCondition=1
  Product : Product  Inputs=*/
  Product1 : Product
  S-Function : S-Function  FunctionName=hysterisis  Parameters=upper,lower  EnableBusSupport=off  mask{upper=upper, lower=lower}
      mask prompts: upper "Upper bound"; lower "Lower bound"
  Saturation : Saturate  UpperLimit=wasteGateMax  LowerLimit=wasteGateMin  mask{max=max, min=min}
      mask prompts: max "Maximum allowable valve opening"; min "Maximum allowable valve opening"
  Sum : Sum  Inputs=|++
  Sum1 : Sum  Inputs=|+-
  Sum2 : Sum  Inputs=|++
  Sum3 : Sum  Inputs=|++
  SumI2 : Sum  DisableCoverage=on  Inputs=-+|
  wasteGateOpen : Outport
  wires:
  S-Function/1 -> Product1/1
  pScav/1 -> S-Function/1
  Gain2/1 -> Gain1/1
  Sum3/1 -> Gain2/1
  Gain3/1 -> Sum3/2
  SumI2/1 -> Gain3/1  "u_sat_error"
  u saturated/1 -> SumI2/2
  Sum2/1 -> SumI2/1, Saturation/1
  Sum1/1 -> Gain/1, Sum3/1
  Gain/1 -> Sum2/1
  Gain1/1 -> Integrator/1
  Integrator/1 -> Sum2/2
  Constant/1 -> Sum/2
  Sum/1 -> Product/2
  Product/1 -> Sum1/2
  Constant1/1 -> Sum1/1
  Saturation/1 -> Product1/2
  Product1/1 -> wasteGateOpen/1
  dmExhBypass/1 -> Product/1
  dmExhTotal/1 -> Sum/1

== matlab function Propeller ==
  data: omegaE input double; Tq output double; coeffProp parameter double
function Tq = propellerLaw(omegaE,coeffProp)
%#codegen
    Tq = ((coeffProp(1)*omegaE + coeffProp(2))*omegaE + coeffProp(3))*1000;
end

== matlab function Shaft/MATLAB Function ==
  data: omegaE input double; effMech output double; omegaEMax parameter double; coeffMechEff parameter double
function effMech = mechEff(omegaE,omegaEMax,coeffMechEff)
%#codegen
	omega_nom = omegaE/omegaEMax;		
	effMech = 1 - (coeffMechEff(2)*omega_nom - (coeffMechEff(1)/ ...
        (1-coeffMechEff(2)))*(omega_nom-coeffMechEff(2))*omega_nom);
end
